simulink model "Prop_VV"  (R2020b)
settings: Solver=VariableStepAuto  StartTime=0.0  StopTime=10.0  RelTol=1e-3
values from neighbouring files (symbols this model uses):
  Fb1_l = -Fulim_BF    (= -26000)    [Prop_V.m]
  Fb1_u = Fulim_BF    (= 26000)    [Prop_V.m]
  Fb2_l = -Fulim_BF    (= -26000)    [Prop_V.m]
  Fb2_u = Fulim_BF    (= 26000)    [Prop_V.m]
  Fb3_l = -Fulim_Back    (= -32000)    [Prop_V.m]
  Fb3_u = Fulim_Back    (= 32000)    [Prop_V.m]
  Fb4_l = -Fulim_Back    (= -32000)    [Prop_V.m]
  Fb4_u = Fulim_Back    (= 32000)    [Prop_V.m]
  Fc = [F_c1; F_c2; F_c3]    [Prop_V.m]
  Fc1_l = -Fclim    (= -3000)    [Prop_V.m]
  Fc1_u = Fclim    (= 3000)    [Prop_V.m]
  Fc2_l = -Fclim    (= -3000)    [Prop_V.m]
  Fc2_u = Fclim    (= 3000)    [Prop_V.m]
  Fc3_l = -Fclim    (= -3000)    [Prop_V.m]
  Fc3_u = Fclim    (= 3000)    [Prop_V.m]
  fprop = 1000    [Prop_V.m]
  Ft1_l = -Fulim_TF    (= -56000)    [Prop_V.m]
  Ft1_u = Fulim_TF    (= 56000)    [Prop_V.m]
  Ft2_l = -Fulim_TF    (= -56000)    [Prop_V.m]
  Ft2_u = Fulim_TF    (= 56000)    [Prop_V.m]
  Ft3_l = -Fulim_Back    (= -32000)    [Prop_V.m]
  Ft3_u = Fulim_Back    (= 32000)    [Prop_V.m]
  Ft4_l = -Fulim_Back    (= -32000)    [Prop_V.m]
  Ft4_u = Fulim_Back    (= 32000)    [Prop_V.m]
  Mc = rand(3,1)    [Prop_V.m]
  Tdv = [1 0 0 ... (first row only)    [Prop_V.m]
  Tvd = transpose(Tdv)    [Prop_V.m]
libraries: dspsigops x11
settings Model: Creator=Jonathan van Zyl  LastModifiedBy=Jonathan van Zyl

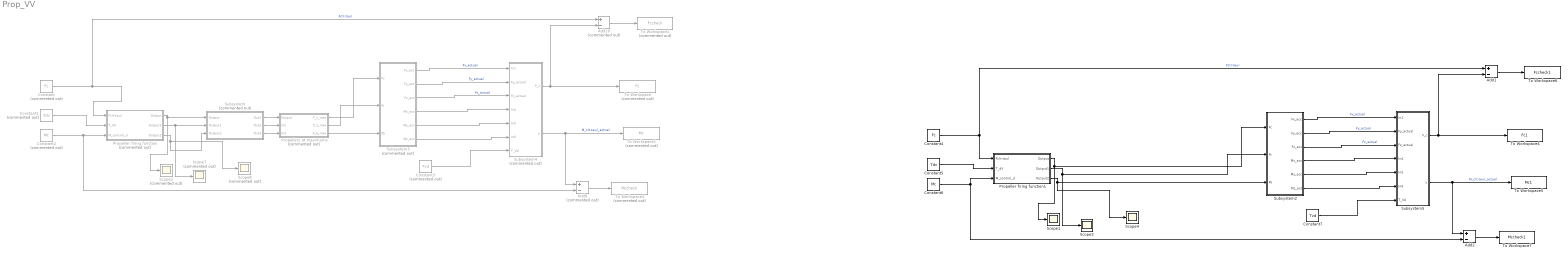
== system Prop_VV ==
  Add1 : Sum  Inputs=+-
  Add10 : Sum  Commented=on  Inputs=+-
  Add2 : Sum  Inputs=+-
  Add9 : Sum  Commented=on  Inputs=+-
  Constant : Constant  Commented=on  Value=Fc
  Constant1 : Constant  Commented=on  Value=Tdv
  Constant2 : Constant  Commented=on  Value=Mc
  Constant3 : Constant  Commented=on  Value=Tvd
  Constant4 : Constant  Value=Fc
  Constant5 : Constant  Value=Tdv
  Constant6 : Constant  Value=Mc
  Constant7 : Constant  Value=Tvd
  Propeller firing function : Subsystem  Commented=on
  Propeller firing function1 : Subsystem
  Propellers at maximums : Subsystem  Commented=on
  Scope1 : Scope
  Scope2 : Scope  Commented=on
  Scope3 : Scope
  Scope4 : Scope
  Scope7 : Scope  Commented=on
  Scope8 : Scope  Commented=on
  Subsystem : Subsystem  Commented=on
  Subsystem2 : Subsystem
  Subsystem3 : Subsystem  Commented=on
  Subsystem4 : Subsystem  Commented=on
  Subsystem5 : Subsystem
  To Workspace : ToWorkspace  Commented=on  VariableName=Fc  SaveFormat=Timeseries  SampleTime=-1
  To Workspace1 : ToWorkspace  Commented=on  VariableName=Mc  SaveFormat=Timeseries  SampleTime=-1
  To Workspace2 : ToWorkspace  Commented=on  VariableName=Fccheck  SaveFormat=Timeseries  SampleTime=-1
  To Workspace3 : ToWorkspace  Commented=on  VariableName=Mccheck  SaveFormat=Timeseries  SampleTime=-1
  To Workspace4 : ToWorkspace  VariableName=Fc1  SaveFormat=Timeseries  SampleTime=-1
  To Workspace5 : ToWorkspace  VariableName=Mc1  SaveFormat=Timeseries  SampleTime=-1
  To Workspace6 : ToWorkspace  VariableName=Fccheck1  SaveFormat=Timeseries  SampleTime=-1
  To Workspace7 : ToWorkspace  VariableName=Mccheck1  SaveFormat=Timeseries  SampleTime=-1
  wires:
  Subsystem/3(Out3) -> Propellers at maximums/3(In3)
  Subsystem/2(Out2) -> Propellers at maximums/2(In2)
  Subsystem/1(Out1) -> Propellers at maximums/1(Output)
  Constant2/1 -> Add9/2, Propeller firing function/3(M_control_d)
  Subsystem3/4(Mx_acc) -> Subsystem4/4(In4)
  Constant3/1 -> Subsystem4/7(T_Vd)
  Constant/1 -> Propeller firing function/1(Fc(t-tau)), Add10/1  "Fc(t-tau)"
  Subsystem4/2(y) -> Add9/1, To Workspace1/1  "M_c(t-tau)_actual"
  Subsystem3/6(Mz_acc) -> Subsystem4/6(In6)
  Subsystem3/5(My_acc) -> Subsystem4/5(In5)
  Subsystem3/1(Fx_acc) -> Subsystem4/1(In1)  "Fx_actual"
  Constant1/1 -> Propeller firing function/2(T_dV)
  Subsystem3/3(Fz_acc) -> Subsystem4/3(Fz_actual)  "Fz_actual"
  Subsystem4/1(F_c) -> To Workspace/1, Add10/2
  Subsystem3/2(Fy_acc) -> Subsystem4/2(Fy_actual)  "Fy_actual"
  Propeller firing function/1(Output) -> Subsystem/1(Output), Scope2/1
  Propeller firing function/2(Output1) -> Scope7/1, Subsystem/2(Output1)
  Propeller firing function/3(Output2) -> Subsystem/3(Output2), Scope8/1
  Add10/1 -> To Workspace2/1
  Add9/1 -> To Workspace3/1
  Propellers at maximums/1(F_c_max) -> Subsystem3/1(Fc)
  Propellers at maximums/2(F_t_max) -> Subsystem3/2(Ft)
  Propellers at maximums/3(F_b_max) -> Subsystem3/3(Fb)
  Propeller firing function1/1(Output) -> Subsystem2/1(Fc), Scope1/1
  Constant6/1 -> Add2/2, Propeller firing function1/3(M_control_d)
  Add2/1 -> To Workspace7/1
  Add1/1 -> To Workspace6/1
  Constant7/1 -> Subsystem5/7(T_Vd)
  Subsystem5/2(y) -> Add2/1, To Workspace5/1  "M_c(t-tau)_actual"
  Subsystem2/2(Fy_acc) -> Subsystem5/2(Fy_actual)  "Fy_actual"
  Subsystem5/1(F_c) -> To Workspace4/1, Add1/2
  Subsystem2/3(Fz_acc) -> Subsystem5/3(Fz_actual)  "Fz_actual"
  Subsystem2/1(Fx_acc) -> Subsystem5/1(In1)  "Fx_actual"
  Subsystem2/4(Mx_acc) -> Subsystem5/4(In4)
  Propeller firing function1/3(Output2) -> Scope4/1, Subsystem2/3(Fb)
  Constant5/1 -> Propeller firing function1/2(T_dV)
  Subsystem2/5(My_acc) -> Subsystem5/5(In5)
  Constant4/1 -> Propeller firing function1/1(Fc(t-tau)), Add1/1  "Fc(t-tau)"
  Propeller firing function1/2(Output1) -> Subsystem2/2(Ft), Scope3/1
  Subsystem2/6(Mz_acc) -> Subsystem5/6(In6)

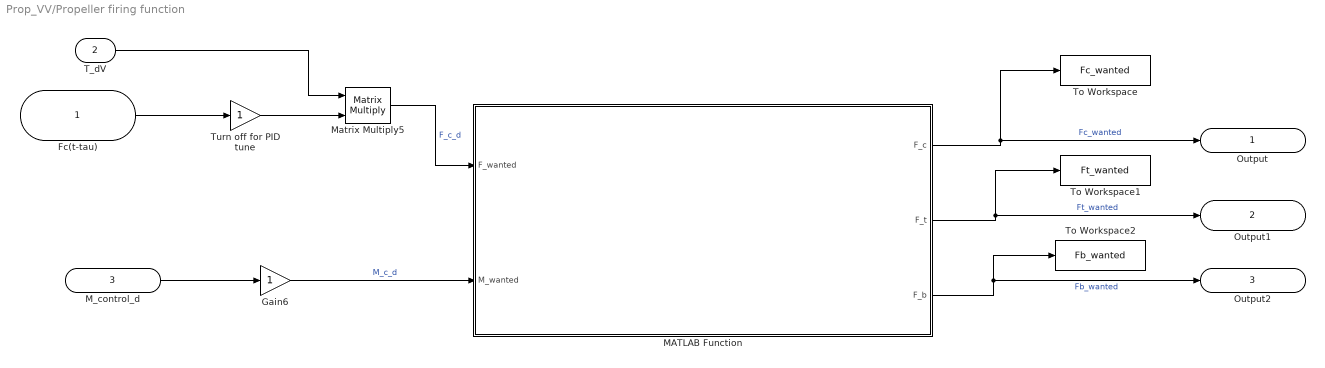
== system Prop_VV/Propeller firing function ==
  Fc(t-tau) : Inport
  T_dV : Inport  Port=2
  M_control_d : Inport  Port=3
  Gain6 : Gain
  MATLAB Function : MATLAB Function  TreatAsAtomicUnit=on
  Matrix Multiply5 : Product  Multiplication=Matrix(*)
  To Workspace : ToWorkspace  VariableName=Fc_wanted  SaveFormat=Timeseries  SampleTime=-1
  To Workspace1 : ToWorkspace  VariableName=Ft_wanted  SaveFormat=Timeseries  SampleTime=-1
  To Workspace2 : ToWorkspace  VariableName=Fb_wanted  SaveFormat=Timeseries  SampleTime=-1
  Turn off for PID tune : Gain
  Output : Outport
  Output1 : Outport  Port=2
  Output2 : Outport  Port=3
  wires:
  Turn off for PID tune/1 -> Matrix Multiply5/2
  Fc(t-tau)/1 -> Turn off for PID tune/1
  Matrix Multiply5/1 -> MATLAB Function/1(F_wanted)  "F_c_d"
  M_control_d/1 -> Gain6/1
  Gain6/1 -> MATLAB Function/2(M_wanted)  "M_c_d"
  MATLAB Function/2(F_t) -> To Workspace1/1, Output1/1  "Ft_wanted"
  MATLAB Function/3(F_b) -> Output2/1, To Workspace2/1  "Fb_wanted"
  MATLAB Function/1(F_c) -> To Workspace/1, Output/1  "Fc_wanted"
  T_dV/1 -> Matrix Multiply5/1

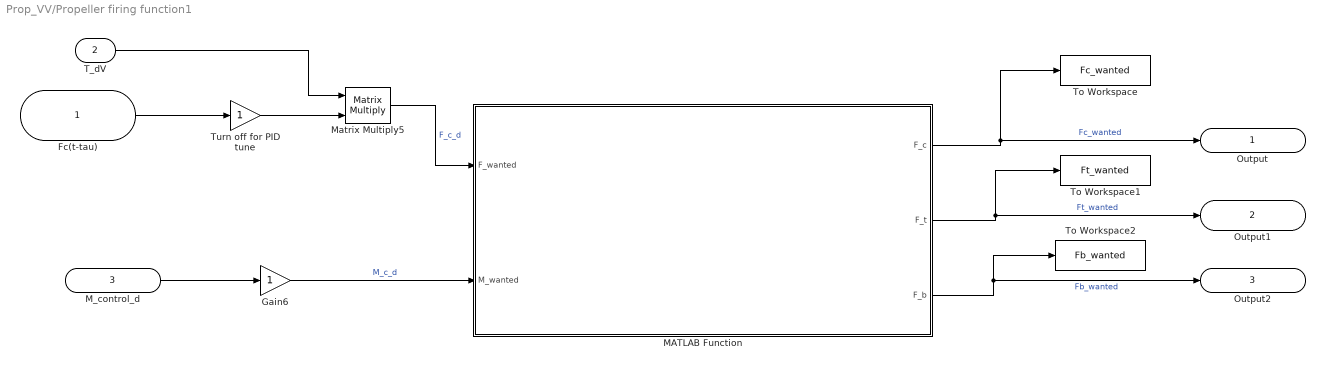
== system Prop_VV/Propeller firing function1 ==
  Fc(t-tau) : Inport
  T_dV : Inport  Port=2
  M_control_d : Inport  Port=3
  Gain6 : Gain
  MATLAB Function : MATLAB Function  TreatAsAtomicUnit=on
  Matrix Multiply5 : Product  Multiplication=Matrix(*)
  To Workspace : ToWorkspace  VariableName=Fc_wanted  SaveFormat=Timeseries  SampleTime=-1
  To Workspace1 : ToWorkspace  VariableName=Ft_wanted  SaveFormat=Timeseries  SampleTime=-1
  To Workspace2 : ToWorkspace  VariableName=Fb_wanted  SaveFormat=Timeseries  SampleTime=-1
  Turn off for PID tune : Gain
  Output : Outport
  Output1 : Outport  Port=2
  Output2 : Outport  Port=3
  wires:
  Turn off for PID tune/1 -> Matrix Multiply5/2
  Fc(t-tau)/1 -> Turn off for PID tune/1
  Matrix Multiply5/1 -> MATLAB Function/1(F_wanted)  "F_c_d"
  M_control_d/1 -> Gain6/1
  Gain6/1 -> MATLAB Function/2(M_wanted)  "M_c_d"
  MATLAB Function/2(F_t) -> To Workspace1/1, Output1/1  "Ft_wanted"
  MATLAB Function/3(F_b) -> Output2/1, To Workspace2/1  "Fb_wanted"
  MATLAB Function/1(F_c) -> To Workspace/1, Output/1  "Fc_wanted"
  T_dV/1 -> Matrix Multiply5/1

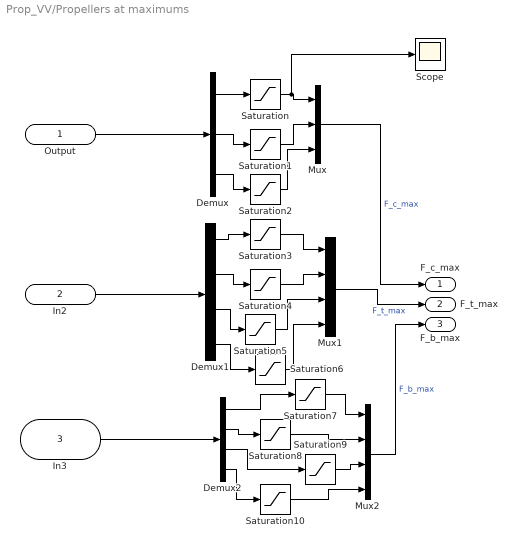
== system Prop_VV/Propellers at maximums ==
  Output : Inport
  In2 : Inport  Port=2
  In3 : Inport  Port=3
  Demux : Demux  Outputs=3
  Demux1 : Demux
  Demux2 : Demux
  Mux : Mux  Inputs=3
  Mux1 : Mux
  Mux2 : Mux
  Saturation : Saturate  UpperLimit=Fc1_u  LowerLimit=Fc1_l
  Saturation1 : Saturate  UpperLimit=Fc2_u  LowerLimit=Fc2_l
  Saturation10 : Saturate  UpperLimit=Fb4_u  LowerLimit=Fb4_l
  Saturation2 : Saturate  UpperLimit=Fc3_u  LowerLimit=Fc3_l
  Saturation3 : Saturate  UpperLimit=Ft1_u  LowerLimit=Ft1_l
  Saturation4 : Saturate  UpperLimit=Ft2_u  LowerLimit=Ft2_l
  Saturation5 : Saturate  UpperLimit=Ft3_u  LowerLimit=Ft3_l
  Saturation6 : Saturate  UpperLimit=Ft4_u  LowerLimit=Ft4_l
  Saturation7 : Saturate  UpperLimit=Fb1_u  LowerLimit=Fb1_l
  Saturation8 : Saturate  UpperLimit=Fb2_u  LowerLimit=Fb2_l
  Saturation9 : Saturate  UpperLimit=Fb3_u  LowerLimit=Fb3_l
  Scope : Scope
  F_c_max : Outport
  F_t_max : Outport  Port=2
  F_b_max : Outport  Port=3
  wires:
  Demux2/1 -> Saturation7/1
  Output/1 -> Demux/1
  Saturation2/1 -> Mux/3
  Mux2/1 -> F_b_max/1  "F_b_max"
  Demux2/2 -> Saturation8/1
  Demux/1 -> Saturation/1
  Demux/2 -> Saturation1/1
  Demux2/3 -> Saturation9/1
  Demux1/1 -> Saturation3/1
  Saturation3/1 -> Mux1/1
  Saturation7/1 -> Mux2/1
  Demux1/4 -> Saturation6/1
  Demux2/4 -> Saturation10/1
  Saturation6/1 -> Mux1/4
  Mux/1 -> F_c_max/1  "F_c_max"
  Saturation/1 -> Scope/1, Mux/1
  Saturation1/1 -> Mux/2
  Mux1/1 -> F_t_max/1  "F_t_max"
  Saturation5/1 -> Mux1/3
  Demux/3 -> Saturation2/1
  Saturation4/1 -> Mux1/2
  Demux1/2 -> Saturation4/1
  Demux1/3 -> Saturation5/1
  Saturation8/1 -> Mux2/2
  Saturation9/1 -> Mux2/3
  Saturation10/1 -> Mux2/4
  In3/1 -> Demux2/1
  In2/1 -> Demux1/1

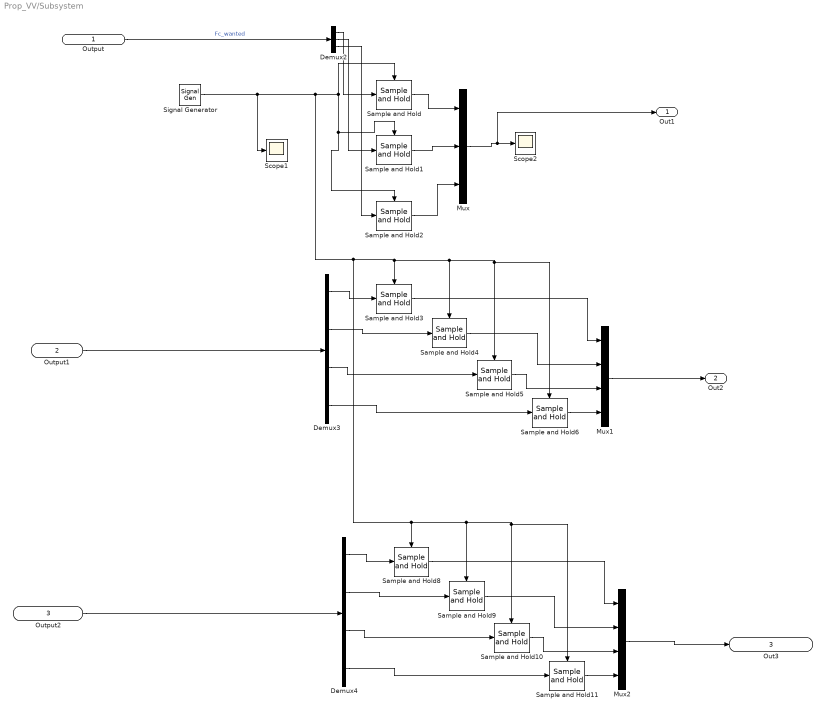
== system Prop_VV/Subsystem ==
  Output : Inport
  Output1 : Inport  Port=2
  Output2 : Inport  Port=3
  Demux2 : Demux  Outputs=3
  Demux3 : Demux
  Demux4 : Demux
  Mux : Mux  Inputs=3
  Mux1 : Mux
  Mux2 : Mux
  Sample and Hold{,1..6,8..11} (11 alike) : dspsigops/Sample and Hold  trig=Rising edge  initCond=0  latchinput=off
  Scope1 : Scope
  Scope2 : Scope
  Signal Generator : SignalGenerator  WaveForm=square  Frequency=fprop  Units=rad/sec
  Out1 : Outport
  Out2 : Outport  Port=2
  Out3 : Outport  Port=3
  wires:
  Sample and Hold/1 -> Mux/1
  Sample and Hold11/1 -> Mux2/4
  Demux2/2 -> Sample and Hold1/1
  Signal Generator/1 -> Scope1/1, Sample and Hold11/Trigger, Sample and Hold10/Trigger, Sample and Hold9/Trigger, Sample and Hold8/Trigger, Sample and Hold6/Trigger, Sample and Hold5/Trigger, Sample and Hold4/Trigger, Sample and Hold3/Trigger, Sample and Hold/Trigger, Sample and Hold2/Trigger, Sample and Hold1/Trigger
  Demux2/3 -> Sample and Hold2/1
  Sample and Hold8/1 -> Mux2/1
  Sample and Hold1/1 -> Mux/2
  Sample and Hold4/1 -> Mux1/2
  Demux2/1 -> Sample and Hold/1
  Output1/1 -> Demux3/1
  Mux/1 -> Out1/1, Scope2/1
  Sample and Hold2/1 -> Mux/3
  Sample and Hold6/1 -> Mux1/4
  Sample and Hold5/1 -> Mux1/3
  Demux3/3 -> Sample and Hold5/1
  Demux3/1 -> Sample and Hold3/1
  Demux3/2 -> Sample and Hold4/1
  Mux2/1 -> Out3/1
  Demux3/4 -> Sample and Hold6/1
  Sample and Hold3/1 -> Mux1/1
  Demux4/2 -> Sample and Hold9/1
  Sample and Hold9/1 -> Mux2/2
  Demux4/1 -> Sample and Hold8/1
  Demux4/4 -> Sample and Hold11/1
  Output/1 -> Demux2/1  "Fc_wanted"
  Demux4/3 -> Sample and Hold10/1
  Sample and Hold10/1 -> Mux2/3
  Output2/1 -> Demux4/1
  Mux1/1 -> Out2/1

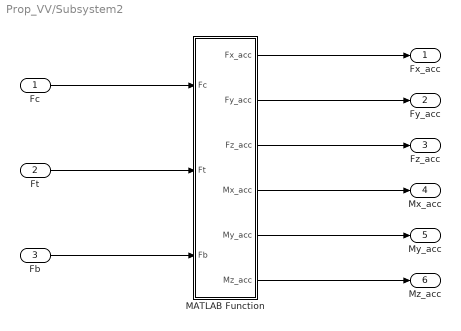
== system Prop_VV/Subsystem2 ==
  Fc : Inport
  Ft : Inport  Port=2
  Fb : Inport  Port=3
  MATLAB Function : MATLAB Function  TreatAsAtomicUnit=on
  Fx_acc : Outport
  Fy_acc : Outport  Port=2
  Fz_acc : Outport  Port=3
  Mx_acc : Outport  Port=4
  My_acc : Outport  Port=5
  Mz_acc : Outport  Port=6
  wires:
  Fc/1 -> MATLAB Function/1(Fc)
  Ft/1 -> MATLAB Function/2(Ft)
  Fb/1 -> MATLAB Function/3(Fb)
  MATLAB Function/1(Fx_acc) -> Fx_acc/1
  MATLAB Function/2(Fy_acc) -> Fy_acc/1
  MATLAB Function/3(Fz_acc) -> Fz_acc/1
  MATLAB Function/4(Mx_acc) -> Mx_acc/1
  MATLAB Function/5(My_acc) -> My_acc/1
  MATLAB Function/6(Mz_acc) -> Mz_acc/1

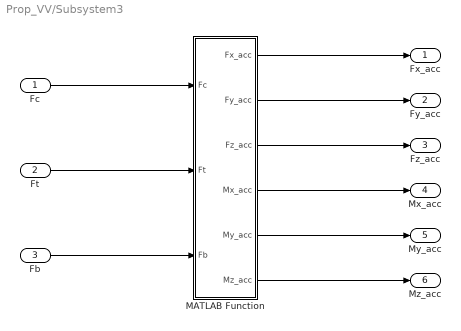
== system Prop_VV/Subsystem3 ==
  Fc : Inport
  Ft : Inport  Port=2
  Fb : Inport  Port=3
  MATLAB Function : MATLAB Function  TreatAsAtomicUnit=on
  Fx_acc : Outport
  Fy_acc : Outport  Port=2
  Fz_acc : Outport  Port=3
  Mx_acc : Outport  Port=4
  My_acc : Outport  Port=5
  Mz_acc : Outport  Port=6
  wires:
  Fc/1 -> MATLAB Function/1(Fc)
  Ft/1 -> MATLAB Function/2(Ft)
  Fb/1 -> MATLAB Function/3(Fb)
  MATLAB Function/1(Fx_acc) -> Fx_acc/1
  MATLAB Function/2(Fy_acc) -> Fy_acc/1
  MATLAB Function/3(Fz_acc) -> Fz_acc/1
  MATLAB Function/4(Mx_acc) -> Mx_acc/1
  MATLAB Function/5(My_acc) -> My_acc/1
  MATLAB Function/6(Mz_acc) -> Mz_acc/1

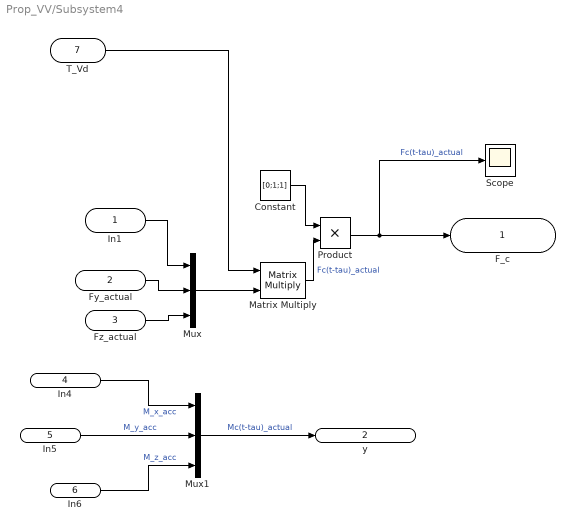
== system Prop_VV/Subsystem4 ==
  In1 : Inport
  Fy_actual : Inport  Port=2
  Fz_actual : Inport  Port=3
  In4 : Inport  Port=4
  In5 : Inport  Port=5
  In6 : Inport  Port=6
  T_Vd : Inport  Port=7
  Constant : Constant  Value=[0;1;1]
  Matrix Multiply : Product  Multiplication=Matrix(*)
  Mux : Mux  Inputs=3
  Mux1 : Mux  Inputs=3
  Product : Product
  Scope : Scope
  F_c : Outport
  y : Outport  Port=2
  wires:
  In1/1 -> Mux/1
  Fy_actual/1 -> Mux/2
  Fz_actual/1 -> Mux/3
  Product/1 -> Scope/1, F_c/1  "Fc(t-tau)_actual"
  Mux/1 -> Matrix Multiply/2
  Mux1/1 -> y/1  "Mc(t-tau)_actual"
  In4/1 -> Mux1/1  "M_x_acc"
  In5/1 -> Mux1/2  "M_y_acc"
  In6/1 -> Mux1/3  "M_z_acc"
  T_Vd/1 -> Matrix Multiply/1
  Constant/1 -> Product/1
  Matrix Multiply/1 -> Product/2  "Fc(t-tau)_actual"

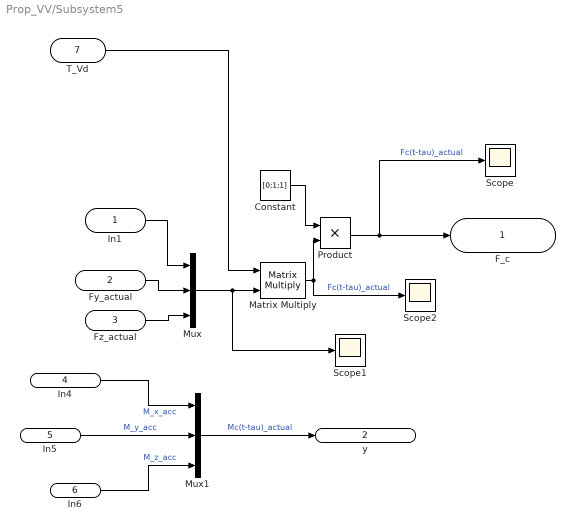
== system Prop_VV/Subsystem5 ==
  In1 : Inport
  Fy_actual : Inport  Port=2
  Fz_actual : Inport  Port=3
  In4 : Inport  Port=4
  In5 : Inport  Port=5
  In6 : Inport  Port=6
  T_Vd : Inport  Port=7
  Constant : Constant  Value=[0;1;1]
  Matrix Multiply : Product  Multiplication=Matrix(*)
  Mux : Mux  Inputs=3
  Mux1 : Mux  Inputs=3
  Product : Product
  Scope : Scope
  Scope1 : Scope
  Scope2 : Scope
  F_c : Outport
  y : Outport  Port=2
  wires:
  In1/1 -> Mux/1
  Fy_actual/1 -> Mux/2
  Fz_actual/1 -> Mux/3
  Product/1 -> Scope/1, F_c/1  "Fc(t-tau)_actual"
  Mux/1 -> Scope1/1, Matrix Multiply/2
  Mux1/1 -> y/1  "Mc(t-tau)_actual"
  In4/1 -> Mux1/1  "M_x_acc"
  In5/1 -> Mux1/2  "M_y_acc"
  In6/1 -> Mux1/3  "M_z_acc"
  T_Vd/1 -> Matrix Multiply/1
  Constant/1 -> Product/1
  Matrix Multiply/1 -> Product/2, Scope2/1  "Fc(t-tau)_actual"

== matlab function Prop_VV/Propeller firing function1/MATLAB Function ==
  data: F_wanted input; F_c output; M_wanted input; F_t output; F_b output
function [F_c, F_t, F_b] = propeller_required_forces_control(F_wanted, M_wanted)

%% New prop arms
%CATIA trans
TcgCatia = [1 0 0;
    0 -1 0;
    0 0 -1];

%Propeller arms - changed due to CATIA errors
t_1 = [1259.8002; 1300; 839.472]*10^(-3);   %Top Front Left
t_2 = [1259.8002; -1300; 839.472]*10^(-3);  %Top Front Right
t_3 = [-1340.1998; 1300; 839.472]*10^(-3);  %Top Back Left
t_4 = [-1340.1998; -1300; 839.472]*10^(-3); %Top Back Right

b_1 = [2259.8002; 1300; -561.25]*10^(-3);   %Bottom Front Left
b_2 = [2259.8002; -1300; -561.25]*10^(-3);  %Bottom Front Right
b_3 = [-1340.1998; 1300; -561.25]*10^(-3);  %Bottom Back Left
b_4 = [-1340.1998; -1300; -561.25]*10^(-3); %Bottom Back Right

c_1 = [-640.1998; 0; 506.566]*10^(-3);      %Control Back Top
c_2 = [-1040.1998; 0; -493.434]*10^(-3);    %Control Back Bottom
c_3 = [2259.8002; 0; -293.434]*10^(-3);     %Control Front

%Propeller arms - rotated
t_1 = TcgCatia*t_1;
t1 = transpose(t_1);
t_2 = TcgCatia*t_2;
t2 = transpose(t_2);
t_3 = TcgCatia*t_3;
t3 = transpose(t_3);
t_4 = TcgCatia*t_4;
t4 = transpose(t_4);
b_1 = TcgCatia*b_1;
b1 = transpose(b_1);
b_2 = TcgCatia*b_2;
b2 = transpose(b_2);
b_3 = TcgCatia*b_3;
b3 = transpose(b_3);
b_4 = TcgCatia*b_4;
b4 = transpose(b_4);
c_1 = TcgCatia*c_1;
c1 = transpose(c_1);
c_2 = TcgCatia*c_2;
c2 = transpose(c_2);
c_3 = TcgCatia*c_3;
c3 = transpose(c_3);

prop_arms = [t1;t2;t3;t4;b1;b2;b3;b4;c1;c2;c3];

props = struct('t1', t1, 't2', t2, 't3', t3, 't4', t4, 'b1', b1, 'b2', b2, 'b3', b3, 'b4', b4, 'c1', c1, 'c2', c2, 'c3', c3);

xc_1 = props.c1(1);
yc_1 = props.c1(2);
zc_1 = props.c1(3);

xc_2 = props.c2(1);
yc_2 = props.c2(2);
zc_2 = props.c2(3);

xc_3 = props.c3(1);
yc_3 = props.c3(2);
zc_3 = props.c3(3);

xt_1 = props.t1(1);
yt_1 = props.t1(2);
zt_1 = props.t1(3);

xt_2 = props.t2(1);
yt_2 = props.t2(2);
zt_2 = props.t2(3);

xt_3 = props.t3(1);
yt_3 = props.t3(2);
zt_3 = props.t3(3);

xt_4 = props.t4(1);
yt_4 = props.t4(2);
zt_4 = props.t4(3);

xb_1 = props.b1(1);
yb_1 = props.b1(2);
zb_1 = props.b1(3);

xb_2 = props.b2(1);
yb_2 = props.b2(2);
zb_2 = props.b2(3);

xb_3 = props.b3(1);
yb_3 = props.b3(2);
zb_3 = props.b3(3);

xb_4 = props.b4(1);
yb_4 = props.b4(2);
zb_4 = props.b4(3);

%% Decompose force and moment input

F_x = F_wanted(1);
F_y = F_wanted(2);

F_z = F_wanted(3);

M_x = M_wanted(1);
M_y = M_wanted(2);
M_z = M_wanted(3);

%% Find control forces
A_control = [1 1 1;
    zc_1 -zc_2 -zc_3;
    -xc_1 -xc_2 xc_3];
A_cinv = inv(A_control);
force_control = [F_y; M_x; M_z];
controlvec = A_cinv*force_control;
F_c1 = controlvec(1);
F_c2 = controlvec(2);
F_c3 = controlvec(3);

%% Find top and bottom forces
A_tb = [-1 -1;
    2*(xt_1 + xb_1) -2*(xt_3 + xb_3)];
A_tbinv = inv(A_tb);
force_tb = [F_z; M_y];
tbvec = A_tbinv * force_tb;
f_front = tbvec(1);
F_t1 = f_front/4;
F_t2 = f_front/4;
F_b1 = f_front/4;
F_b2 = f_front/4;
f_back = tbvec(2);
F_t3 = f_back/4;
F_t4 = f_back/4;
F_b3 = f_back/4;
F_b4 = f_back/4;



%% Make matrix
F_c = [F_c1; F_c2; F_c3];
F_t = [F_t1; F_t2; F_t3; F_t4];
F_b = [F_b1; F_b2; F_b3; F_b4];
end

== matlab function Prop_VV/Subsystem2/MATLAB Function ==
  data: Fc input; Fx_acc output; Ft input; Fb input; Fy_acc output; Fz_acc output; Mx_acc output; My_acc output; Mz_acc output
function [Fx_acc,Fy_acc, Fz_acc, Mx_acc, My_acc, Mz_acc] = fcn(Fc, Ft, Fb)

%% New prop arms
%CATIA trans
TcgCatia = [1 0 0;
    0 -1 0;
    0 0 -1];

%Propeller arms - changed due to CATIA errors
t_1 = [1259.8002; 1300; 839.472]*10^(-3);   %Top Front Left
t_2 = [1259.8002; -1300; 839.472]*10^(-3);  %Top Front Right
t_3 = [-1340.1998; 1300; 839.472]*10^(-3);  %Top Back Left
t_4 = [-1340.1998; -1300; 839.472]*10^(-3); %Top Back Right

b_1 = [2259.8002; 1300; -561.25]*10^(-3);   %Bottom Front Left
b_2 = [2259.8002; -1300; -561.25]*10^(-3);  %Bottom Front Right
b_3 = [-1340.1998; 1300; -561.25]*10^(-3);  %Bottom Back Left
b_4 = [-1340.1998; -1300; -561.25]*10^(-3); %Bottom Back Right

c_1 = [-640.1998; 0; 506.566]*10^(-3);      %Control Back Top
c_2 = [-1040.1998; 0; -493.434]*10^(-3);    %Control Back Bottom
c_3 = [2259.8002; 0; -293.434]*10^(-3);     %Control Front

%Propeller arms - rotated
t_1 = TcgCatia*t_1;
t1 = transpose(t_1);
t_2 = TcgCatia*t_2;
t2 = transpose(t_2);
t_3 = TcgCatia*t_3;
t3 = transpose(t_3);
t_4 = TcgCatia*t_4;
t4 = transpose(t_4);
b_1 = TcgCatia*b_1;
b1 = transpose(b_1);
b_2 = TcgCatia*b_2;
b2 = transpose(b_2);
b_3 = TcgCatia*b_3;
b3 = transpose(b_3);
b_4 = TcgCatia*b_4;
b4 = transpose(b_4);
c_1 = TcgCatia*c_1;
c1 = transpose(c_1);
c_2 = TcgCatia*c_2;
c2 = transpose(c_2);
c_3 = TcgCatia*c_3;
c3 = transpose(c_3);

prop_arms = [t1;t2;t3;t4;b1;b2;b3;b4;c1;c2;c3];

props = struct('t1', t1, 't2', t2, 't3', t3, 't4', t4, 'b1', b1, 'b2', b2, 'b3', b3, 'b4', b4, 'c1', c1, 'c2', c2, 'c3', c3);

xc_1 = props.c1(1);
yc_1 = props.c1(2);
zc_1 = props.c1(3);

xc_2 = props.c2(1);
yc_2 = props.c2(2);
zc_2 = props.c2(3);

xc_3 = props.c3(1);
yc_3 = props.c3(2);
zc_3 = props.c3(3);

xt_1 = props.t1(1);
yt_1 = props.t1(2);
zt_1 = props.t1(3);

xt_2 = props.t2(1);
yt_2 = props.t2(2);
zt_2 = props.t2(3);

xt_3 = props.t3(1);
yt_3 = props.t3(2);
zt_3 = props.t3(3);

xt_4 = props.t4(1);
yt_4 = props.t4(2);
zt_4 = props.t4(3);

xb_1 = props.b1(1);
yb_1 = props.b1(2);
zb_1 = props.b1(3);

xb_2 = props.b2(1);
yb_2 = props.b2(2);
zb_2 = props.b2(3);

xb_3 = props.b3(1);
yb_3 = props.b3(2);
zb_3 = props.b3(3);

xb_4 = props.b4(1);
yb_4 = props.b4(2);
zb_4 = props.b4(3);
%% Split vectors
Fx_acc = 0;

A_control = [1 1 1;
    zc_1 -zc_2 -zc_3;
    -xc_1 -xc_2 xc_3];
ab_control = A_control*Fc;
Fy_acc = ab_control(1);
Mx_acc = ab_control(2);
Mz_acc = ab_control(3);

A_tb = [-1 -1;
    2*(xt_1 + xb_1) -2*(xt_3 + xb_3)];
F_front = Ft(1) + Ft(2) + Fb(1) + Fb(2);
F_back = Ft(3) + Ft(4) + Fb(3) + Fb(4);
Ftb_vec = [F_front; F_back];
Ab_tb = A_tb*Ftb_vec;

Fz_acc = Ab_tb(1);
My_acc = Ab_tb(2);

end

== matlab function Prop_VV/Propeller firing function/MATLAB Function ==
  data: F_wanted input; F_c output; M_wanted input; F_t output; F_b output
function [F_c, F_t, F_b] = propeller_required_forces_control(F_wanted, M_wanted)

%% New prop arms
%CATIA trans
TcgCatia = [1 0 0;
    0 -1 0;
    0 0 -1];

%Propeller arms - changed due to CATIA errors
t_1 = [1259.8002; 1300; 839.472]*10^(-3);   %Top Front Left
t_2 = [1259.8002; -1300; 839.472]*10^(-3);  %Top Front Right
t_3 = [-1340.1998; 1300; 839.472]*10^(-3);  %Top Back Left
t_4 = [-1340.1998; -1300; 839.472]*10^(-3); %Top Back Right

b_1 = [2259.8002; 1300; -561.25]*10^(-3);   %Bottom Front Left
b_2 = [2259.8002; -1300; -561.25]*10^(-3);  %Bottom Front Right
b_3 = [-1340.1998; 1300; -561.25]*10^(-3);  %Bottom Back Left
b_4 = [-1340.1998; -1300; -561.25]*10^(-3); %Bottom Back Right

c_1 = [-640.1998; 0; 506.566]*10^(-3);      %Control Back Top
c_2 = [-1040.1998; 0; -493.434]*10^(-3);    %Control Back Bottom
c_3 = [2259.8002; 0; -293.434]*10^(-3);     %Control Front

%Propeller arms - rotated
t_1 = TcgCatia*t_1;
t1 = transpose(t_1);
t_2 = TcgCatia*t_2;
t2 = transpose(t_2);
t_3 = TcgCatia*t_3;
t3 = transpose(t_3);
t_4 = TcgCatia*t_4;
t4 = transpose(t_4);
b_1 = TcgCatia*b_1;
b1 = transpose(b_1);
b_2 = TcgCatia*b_2;
b2 = transpose(b_2);
b_3 = TcgCatia*b_3;
b3 = transpose(b_3);
b_4 = TcgCatia*b_4;
b4 = transpose(b_4);
c_1 = TcgCatia*c_1;
c1 = transpose(c_1);
c_2 = TcgCatia*c_2;
c2 = transpose(c_2);
c_3 = TcgCatia*c_3;
c3 = transpose(c_3);

prop_arms = [t1;t2;t3;t4;b1;b2;b3;b4;c1;c2;c3];

props = struct('t1', t1, 't2', t2, 't3', t3, 't4', t4, 'b1', b1, 'b2', b2, 'b3', b3, 'b4', b4, 'c1', c1, 'c2', c2, 'c3', c3);

xc_1 = props.c1(1);
yc_1 = props.c1(2);
zc_1 = props.c1(3);

xc_2 = props.c2(1);
yc_2 = props.c2(2);
zc_2 = props.c2(3);

xc_3 = props.c3(1);
yc_3 = props.c3(2);
zc_3 = props.c3(3);

xt_1 = props.t1(1);
yt_1 = props.t1(2);
zt_1 = props.t1(3);

xt_2 = props.t2(1);
yt_2 = props.t2(2);
zt_2 = props.t2(3);

xt_3 = props.t3(1);
yt_3 = props.t3(2);
zt_3 = props.t3(3);

xt_4 = props.t4(1);
yt_4 = props.t4(2);
zt_4 = props.t4(3);

xb_1 = props.b1(1);
yb_1 = props.b1(2);
zb_1 = props.b1(3);

xb_2 = props.b2(1);
yb_2 = props.b2(2);
zb_2 = props.b2(3);

xb_3 = props.b3(1);
yb_3 = props.b3(2);
zb_3 = props.b3(3);

xb_4 = props.b4(1);
yb_4 = props.b4(2);
zb_4 = props.b4(3);

%% Decompose force and moment input

F_x = F_wanted(1);
F_y = F_wanted(2);

F_z = F_wanted(3);

M_x = M_wanted(1);
M_y = M_wanted(2);
M_z = M_wanted(3);

%% Find control forces
A_control = [1 1 1;
    zc_1 -zc_2 -zc_3;
    -xc_1 -xc_2 xc_3];
A_cinv = inv(A_control);
force_control = [F_y; M_x; M_z];
controlvec = A_cinv*force_control;
F_c1 = controlvec(1);
F_c2 = controlvec(2);
F_c3 = controlvec(3);

%% Find top and bottom forces
A_tb = [-1 -1;
    2*(xt_1 + xb_1) -2*(xt_3 + xb_3)];
A_tbinv = inv(A_tb);
force_tb = [F_z; M_y];
tbvec = A_tbinv * force_tb;
f_front = tbvec(1);
F_t1 = f_front/4;
F_t2 = f_front/4;
F_b1 = f_front/4;
F_b2 = f_front/4;
f_back = tbvec(2);
F_t3 = f_back/4;
F_t4 = f_back/4;
F_b3 = f_back/4;
F_b4 = f_back/4;



%% Make matrix
F_c = [F_c1; F_c2; F_c3];
F_t = [F_t1; F_t2; F_t3; F_t4];
F_b = [F_b1; F_b2; F_b3; F_b4];
end

== matlab function Prop_VV/Subsystem3/MATLAB Function ==
  data: Fc input; Fx_acc output; Ft input; Fb input; Fy_acc output; Fz_acc output; Mx_acc output; My_acc output; Mz_acc output
function [Fx_acc,Fy_acc, Fz_acc, Mx_acc, My_acc, Mz_acc] = fcn(Fc, Ft, Fb)

%% New prop arms
%CATIA trans
TcgCatia = [1 0 0;
    0 -1 0;
    0 0 -1];

%Propeller arms - changed due to CATIA errors
t_1 = [1259.8002; 1300; 839.472]*10^(-3);   %Top Front Left
t_2 = [1259.8002; -1300; 839.472]*10^(-3);  %Top Front Right
t_3 = [-1340.1998; 1300; 839.472]*10^(-3);  %Top Back Left
t_4 = [-1340.1998; -1300; 839.472]*10^(-3); %Top Back Right

b_1 = [2259.8002; 1300; -561.25]*10^(-3);   %Bottom Front Left
b_2 = [2259.8002; -1300; -561.25]*10^(-3);  %Bottom Front Right
b_3 = [-1340.1998; 1300; -561.25]*10^(-3);  %Bottom Back Left
b_4 = [-1340.1998; -1300; -561.25]*10^(-3); %Bottom Back Right

c_1 = [-640.1998; 0; 506.566]*10^(-3);      %Control Back Top
c_2 = [-1040.1998; 0; -493.434]*10^(-3);    %Control Back Bottom
c_3 = [2259.8002; 0; -293.434]*10^(-3);     %Control Front

%Propeller arms - rotated
t_1 = TcgCatia*t_1;
t1 = transpose(t_1);
t_2 = TcgCatia*t_2;
t2 = transpose(t_2);
t_3 = TcgCatia*t_3;
t3 = transpose(t_3);
t_4 = TcgCatia*t_4;
t4 = transpose(t_4);
b_1 = TcgCatia*b_1;
b1 = transpose(b_1);
b_2 = TcgCatia*b_2;
b2 = transpose(b_2);
b_3 = TcgCatia*b_3;
b3 = transpose(b_3);
b_4 = TcgCatia*b_4;
b4 = transpose(b_4);
c_1 = TcgCatia*c_1;
c1 = transpose(c_1);
c_2 = TcgCatia*c_2;
c2 = transpose(c_2);
c_3 = TcgCatia*c_3;
c3 = transpose(c_3);

prop_arms = [t1;t2;t3;t4;b1;b2;b3;b4;c1;c2;c3];

props = struct('t1', t1, 't2', t2, 't3', t3, 't4', t4, 'b1', b1, 'b2', b2, 'b3', b3, 'b4', b4, 'c1', c1, 'c2', c2, 'c3', c3);

xc_1 = props.c1(1);
yc_1 = props.c1(2);
zc_1 = props.c1(3);

xc_2 = props.c2(1);
yc_2 = props.c2(2);
zc_2 = props.c2(3);

xc_3 = props.c3(1);
yc_3 = props.c3(2);
zc_3 = props.c3(3);

xt_1 = props.t1(1);
yt_1 = props.t1(2);
zt_1 = props.t1(3);

xt_2 = props.t2(1);
yt_2 = props.t2(2);
zt_2 = props.t2(3);

xt_3 = props.t3(1);
yt_3 = props.t3(2);
zt_3 = props.t3(3);

xt_4 = props.t4(1);
yt_4 = props.t4(2);
zt_4 = props.t4(3);

xb_1 = props.b1(1);
yb_1 = props.b1(2);
zb_1 = props.b1(3);

xb_2 = props.b2(1);
yb_2 = props.b2(2);
zb_2 = props.b2(3);

xb_3 = props.b3(1);
yb_3 = props.b3(2);
zb_3 = props.b3(3);

xb_4 = props.b4(1);
yb_4 = props.b4(2);
zb_4 = props.b4(3);
%% Split vectors
Fx_acc = 0;

A_control = [1 1 1;
    zc_1 -zc_2 -zc_3;
    -xc_1 -xc_2 xc_3];
ab_control = A_control*Fc;
Fy_acc = ab_control(1);
Mx_acc = ab_control(2);
Mz_acc = ab_control(3);

A_tb = [-1 -1;
    2*(xt_1 + xb_1) -2*(xt_3 + xb_3)];
F_front = Ft(1) + Ft(2) + Fb(1) + Fb(2);
F_back = Ft(3) + Ft(4) + Fb(3) + Fb(4);
Ftb_vec = [F_front; F_back];
Ab_tb = A_tb*Ftb_vec;

Fz_acc = Ab_tb(1);
My_acc = Ab_tb(2);

end
